simulink model "controller"  (R2022b)
settings: Solver=VariableStepAuto  StartTime=0.0  StopTime=160  RelTol=1e-3
undefined symbols (not defined in the file or in its folder): SS_glide_A, SS_glide_B, SS_glide_C, SS_glide_D
libraries: simulink_extras x5, cstblocks x2
settings Model: Creator=micky  LastModifiedBy=micky

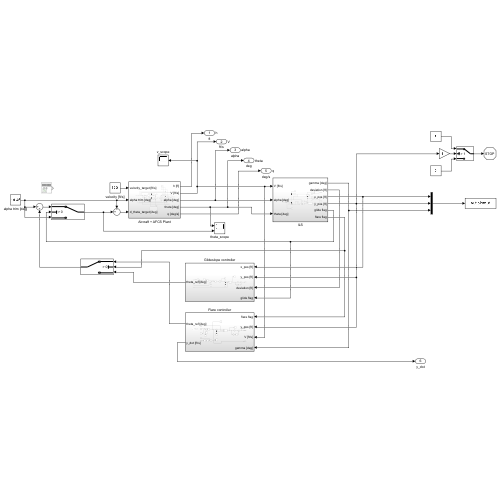
[thumbnail: Simulink's stored preview of the top-level diagram]
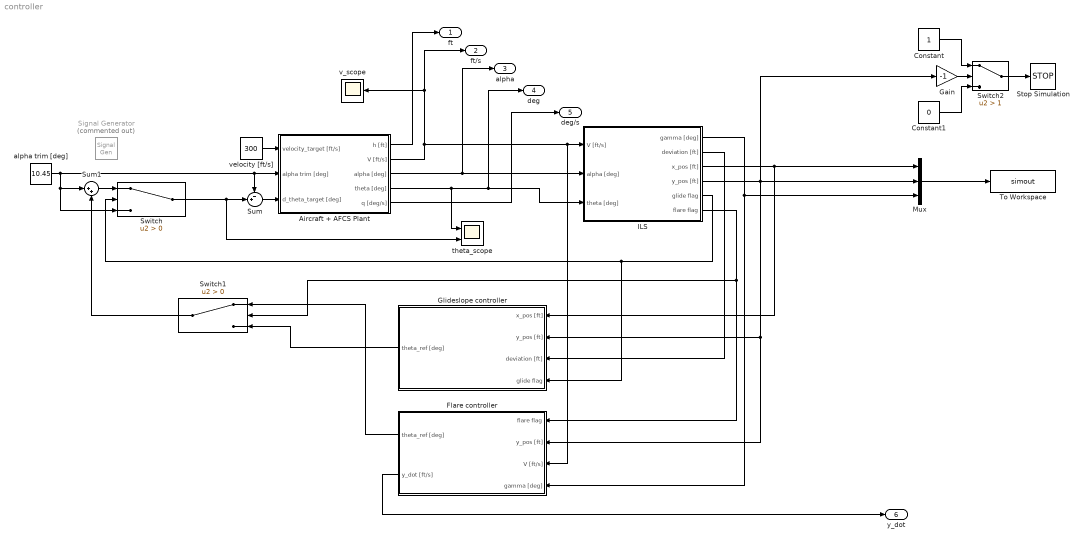
== system controller ==
  Aircraft + AFCS Plant : Subsystem
  Constant : Constant
  Constant1 : Constant  Value=0
  Flare controller : Subsystem
  Gain : Gain  Gain=-1
  Glideslope controller : Subsystem
  ILS : Subsystem
  Mux : Mux  Inputs=3
  Signal Generator : SignalGenerator  Commented=on  WaveForm=square  Frequency=0.6  Units=rad/sec
  Stop Simulation : Stop
  Sum : Sum  Inputs=-+|
  Sum1 : Sum  Inputs=|++
  Switch : Switch  Criteria=u2 > Threshold  SaturateOnIntegerOverflow=off  InputSameDT=off
  Switch1 : Switch  Criteria=u2 > Threshold  SaturateOnIntegerOverflow=off  InputSameDT=off
  Switch2 : Switch  Criteria=u2 > Threshold  Threshold=1  SaturateOnIntegerOverflow=off  InputSameDT=off
  To Workspace : ToWorkspace  VariableName=simout  SaveFormat=Timeseries  SampleTime=-1
  alpha trim [deg] : Constant  Value=10.45
  theta_scope : Scope  NumInputPorts=2
  v_scope : Scope
  velocity [ft/s] : Constant  Value=300
  ft : Outport  SignalName=h
  ft/s : Outport  Port=2  SignalName=V
  alpha : Outport  Port=3  SignalName=alpha
  deg : Outport  Port=4  SignalName=theta
  deg/s : Outport  Port=5  SignalName=q
  y_dot : Outport  Port=6
  wires:
  Aircraft + AFCS Plant/1(h [ft]) -> ft/1
  Aircraft + AFCS Plant/2(V [ft/s]) -> ft/s/1, v_scope/1, ILS/1(V [ft/s]), Flare controller/3(V [ft/s])
  Aircraft + AFCS Plant/3(alpha [deg]) -> alpha/1, ILS/2(alpha [deg])
  Aircraft + AFCS Plant/4(theta [deg]) -> theta_scope/1, ILS/3(theta [deg]), deg/1
  Aircraft + AFCS Plant/5(q [deg/s]) -> deg/s/1
  velocity [ft/s]/1 -> Aircraft + AFCS Plant/1(velocity_target [ft/s])
  ILS/1(gamma [deg]) -> Flare controller/4(gamma [deg]), Mux/3
  ILS/4(y_pos [ft]) -> Gain/1, Mux/2, Glideslope controller/2(y_pos [ft]), Flare controller/2(y_pos [ft])
  ILS/3(x_pos [ft]) -> Glideslope controller/1(x_pos [ft]), Mux/1
  ILS/2(deviation [ft]) -> Glideslope controller/3(deviation [ft])
  alpha trim [deg]/1 -> Sum/1, Aircraft + AFCS Plant/2(alpha trim [deg]), Sum1/1, Switch/3
  Glideslope controller/1(theta_ref [deg]) -> Switch1/3
  Sum/1 -> Aircraft + AFCS Plant/3(d_theta_target [deg])
  Switch/1 -> theta_scope/2, Sum/2
  Mux/1 -> To Workspace/1
  Switch1/1 -> Sum1/2
  Flare controller/1(theta_ref [deg]) -> Switch1/1
  ILS/5(glide flag) -> Glideslope controller/4(glide flag), Switch/2
  ILS/6(flare flag) -> Switch1/2, Flare controller/1(flare flag)
  Gain/1 -> Switch2/2
  Constant/1 -> Switch2/1
  Constant1/1 -> Switch2/3
  Switch2/1 -> Stop Simulation/1
  Flare controller/2(y_dot [ft/s]) -> y_dot/1
  Sum1/1 -> Switch/1

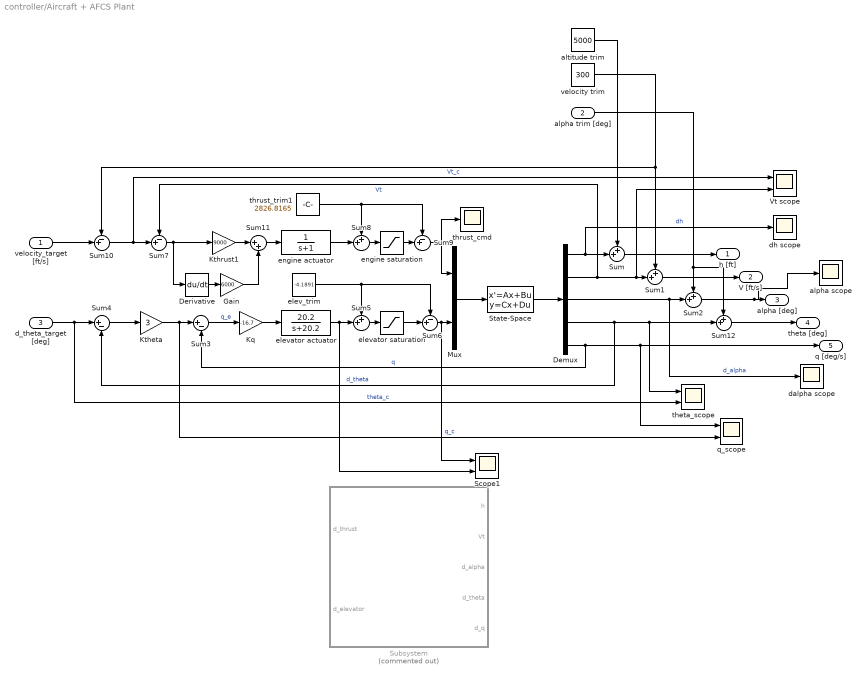
== system controller/Aircraft + AFCS Plant ==
  velocity_target [ft/s] : Inport
  alpha trim [deg] : Inport  Port=2
  d_theta_target [deg] : Inport  Port=3
  Demux : Demux  Outputs=5
  Derivative : Derivative
  Gain : Gain  Gain=6000
  Kq : Gain  Gain=-16.7
  Ktheta : Gain  Gain=3
  Kthrust1 : Gain  Gain=9000
  Mux : Mux  Inputs=2
  Scope1 : Scope  NumInputPorts=2
  State-Space : StateSpace  A=SS_glide_A  B=SS_glide_B  C=SS_glide_C  D=SS_glide_D  InitialCondition=0
  Subsystem : Subsystem  Commented=on
  Sum{,1..2,5,8,12} (6 alike) : Sum  Inputs=++|
  Sum{6..7,9..10} (4 alike) : Sum  Inputs=-+|
  Sum11 : Sum  Inputs=|++
  Sum3 : Sum  Inputs=|+-
  Sum4 : Sum  Inputs=|+-
  Vt scope : Scope  NumInputPorts=2
  alpha scope : Scope
  altitude trim : Constant  Value=5000
  dalpha scope : Scope
  dh scope : Scope
  elev_trim : Constant  Value=-4.1891
  elevator actuator : TransferFcn  Numerator=[20.2]  Denominator=[1 20.2]
  elevator saturation : Saturate  UpperLimit=25  LowerLimit=-25
  engine actuator : TransferFcn  Denominator=[1 1]
  engine saturation : Saturate  UpperLimit=19000  LowerLimit=1000
  q_scope : Scope  NumInputPorts=2
  theta_scope : Scope  NumInputPorts=2
  thrust_cmd : Scope
  thrust_trim1 : Constant  Value=2826.8165
  velocity trim : Constant  Value=300
  h [ft] : Outport
  V [ft/s] : Outport  Port=2
  alpha [deg] : Outport  Port=3
  theta [deg] : Outport  Port=4
  q [deg/s] : Outport  Port=5
  wires:
  engine actuator/1 -> Sum8/2
  Sum1/1 -> V [ft/s]/1
  Demux/5 -> Sum3/2, q [deg/s]/1, q_scope/1  "q"
  thrust_trim1/1 -> Sum9/1, Sum8/1
  Sum3/1 -> Kq/1  "q_e"
  Gain/1 -> Sum11/2
  Sum6/1 -> Scope1/1, Mux/2
  velocity_target [ft/s]/1 -> Sum10/2
  altitude trim/1 -> Sum/1
  Demux/3 -> dalpha scope/1, Sum2/2  "d_alpha"
  Kthrust1/1 -> Sum11/1
  Demux/2 -> Vt scope/2, Sum1/2, Sum7/1  "Vt"
  velocity trim/1 -> Sum10/1, Sum1/1
  Sum/1 -> h [ft]/1
  Sum10/1 -> Sum7/2, Vt scope/1  "Vt_c"
  State-Space/1 -> Demux/1
  Demux/4 -> Sum12/2, theta_scope/1, Sum4/2  "d_theta"
  Demux/1 -> dh scope/1, Sum/2  "dh"
  elev_trim/1 -> Sum6/1, Sum5/1
  Mux/1 -> State-Space/1
  Sum7/1 -> Kthrust1/1, Derivative/1
  Ktheta/1 -> q_scope/2, Sum3/1  "q_c"
  Sum4/1 -> Ktheta/1
  d_theta_target [deg]/1 -> theta_scope/2, Sum4/1  "theta_c"
  Sum2/1 -> alpha scope/1, alpha [deg]/1
  Sum5/1 -> elevator saturation/1
  Sum9/1 -> thrust_cmd/1, Mux/1
  Derivative/1 -> Gain/1
  engine saturation/1 -> Sum9/2
  Sum8/1 -> engine saturation/1
  elevator saturation/1 -> Sum6/2
  Kq/1 -> elevator actuator/1
  elevator actuator/1 -> Scope1/2, Sum5/2
  Sum11/1 -> engine actuator/1
  Sum12/1 -> theta [deg]/1
  alpha trim [deg]/1 -> Sum12/1, Sum2/1

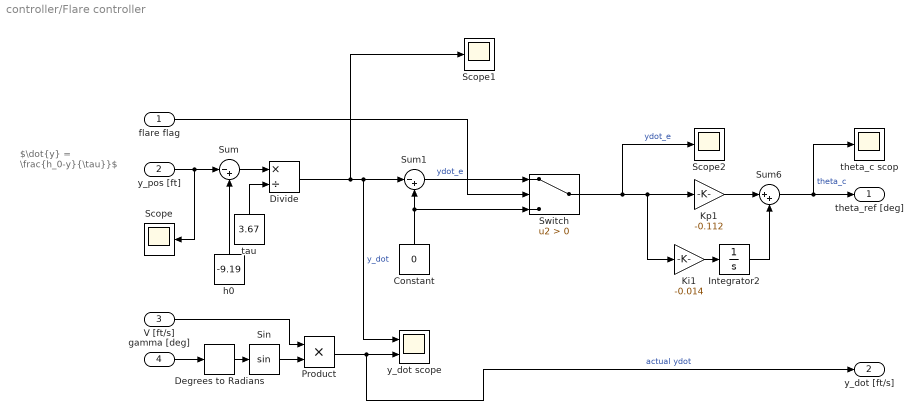
== system controller/Flare controller ==
  note: $\dot{y} = \frac{h_0-y}{\tau}}$
  flare flag : Inport
  y_pos [ft] : Inport  Port=2
  V [ft/s] : Inport  Port=3
  gamma [deg] : Inport  Port=4
  Constant : Constant  Value=0
  Degrees to Radians : simulink_extras/Transformations/Degrees to Radians
  Divide : Product  Inputs=*/
  Integrator2 : Integrator
  Ki1 : Gain  Gain=-0.014
  Kp1 : Gain  Gain=-0.112
  Product : Product
  Scope : Scope
  Scope1 : Scope
  Scope2 : Scope
  Sin : Trigonometry
  Sum : Sum  Inputs=|-+
  Sum1 : Sum  Inputs=|-+
  Sum6 : Sum  Inputs=|++
  Switch : Switch  Criteria=u2 > Threshold  SaturateOnIntegerOverflow=off  InputSameDT=off
  h0 : Constant  Value=-9.19
  tau : Constant  Value=3.67
  theta_c scop : Scope
  y_dot scope : Scope  NumInputPorts=2
  theta_ref [deg] : Outport
  y_dot [ft/s] : Outport  Port=2
  wires:
  h0/1 -> Sum/2
  y_pos [ft]/1 -> Sum/1, Scope/1
  Sum/1 -> Divide/1
  tau/1 -> Divide/2
  Divide/1 -> Scope1/1, Sum1/1, y_dot scope/1  "y_dot"
  gamma [deg]/1 -> Degrees to Radians/1
  Degrees to Radians/1 -> Sin/1
  Sin/1 -> Product/2
  V [ft/s]/1 -> Product/1
  Product/1 -> y_dot [ft/s]/1, y_dot scope/2  "actual ydot"
  Sum1/1 -> Switch/1  "ydot_e"
  Sum6/1 -> theta_c scop/1, theta_ref [deg]/1  "theta_c"
  Kp1/1 -> Sum6/1
  Switch/1 -> Scope2/1, Kp1/1, Ki1/1  "ydot_e"
  Ki1/1 -> Integrator2/1
  flare flag/1 -> Switch/2
  Constant/1 -> Switch/3, Sum1/2
  Integrator2/1 -> Sum6/2

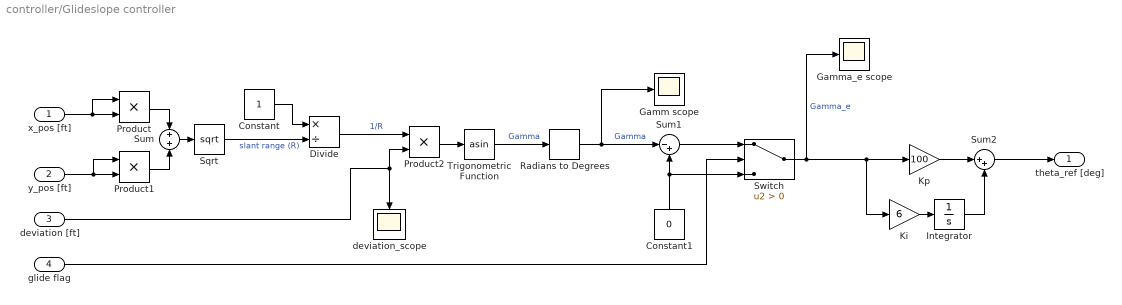
== system controller/Glideslope controller ==
  x_pos [ft] : Inport
  y_pos [ft] : Inport  Port=2
  deviation [ft] : Inport  Port=3
  glide flag : Inport  Port=4
  Constant : Constant
  Constant1 : Constant  Value=0
  Divide : Product  Inputs=*/
  Gamm scope : Scope
  Gamma_e scope : Scope
  Integrator : Integrator
  Ki : Gain  Gain=6
  Kp : Gain  Gain=100
  Product : Product
  Product1 : Product
  Product2 : Product
  Radians to Degrees : simulink_extras/Transformations/Radians to Degrees
  Sqrt : Sqrt
  Sum : Sum
  Sum1 : Sum  Inputs=|-+
  Sum2 : Sum  Inputs=|++
  Switch : Switch  Criteria=u2 > Threshold  SaturateOnIntegerOverflow=off  InputSameDT=off
  Trigonometric Function : Trigonometry  Operator=asin
  deviation_scope : Scope
  theta_ref [deg] : Outport
  wires:
  x_pos [ft]/1 -> Product/2, Product/1
  y_pos [ft]/1 -> Product1/1, Product1/2
  Product/1 -> Sum/1
  Product1/1 -> Sum/2
  Sum/1 -> Sqrt/1
  Sqrt/1 -> Divide/2  "slant range (R)"
  Constant/1 -> Divide/1
  Divide/1 -> Product2/1  "1/R"
  deviation [ft]/1 -> Product2/2, deviation_scope/1
  Product2/1 -> Trigonometric Function/1
  Switch/1 -> Kp/1, Ki/1, Gamma_e scope/1  "Gamma_e"
  Kp/1 -> Sum2/1
  Ki/1 -> Integrator/1
  Integrator/1 -> Sum2/2
  Sum2/1 -> theta_ref [deg]/1
  Radians to Degrees/1 -> Gamm scope/1, Sum1/1  "Gamma"
  glide flag/1 -> Switch/2
  Constant1/1 -> Switch/3, Sum1/2
  Sum1/1 -> Switch/1
  Trigonometric Function/1 -> Radians to Degrees/1  "Gamma"

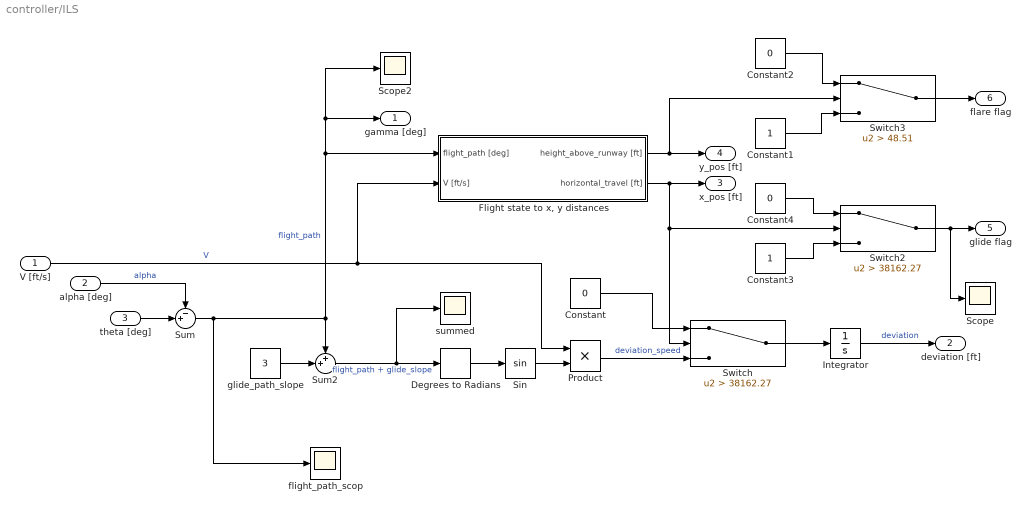
== system controller/ILS ==
  V [ft/s] : Inport
  alpha [deg] : Inport  Port=2
  theta [deg] : Inport  Port=3
  Constant : Constant  Value=0
  Constant1 : Constant
  Constant2 : Constant  Value=0
  Constant3 : Constant
  Constant4 : Constant  Value=0
  Degrees to Radians : simulink_extras/Transformations/Degrees to Radians
  "Flight state to x, y distances" : Subsystem
  Integrator : Integrator
  Product : Product
  Scope : Scope
  Scope2 : Scope
  Sin : Trigonometry
  Sum : Sum  Inputs=-+|
  Sum2 : Sum  Inputs=++|
  Switch : Switch  Criteria=u2 > Threshold  Threshold=38162.27  SaturateOnIntegerOverflow=off  InputSameDT=off
  Switch2 : Switch  Criteria=u2 > Threshold  Threshold=38162.27  SaturateOnIntegerOverflow=off  InputSameDT=off
  Switch3 : Switch  Criteria=u2 > Threshold  Threshold=48.51  SaturateOnIntegerOverflow=off  InputSameDT=off
  flight_path_scop : Scope
  glide_path_slope : Constant  Value=3
  summed : Scope
  gamma [deg] : Outport
  deviation [ft] : Outport  Port=2
  x_pos [ft] : Outport  Port=3
  y_pos [ft] : Outport  Port=4
  glide flag : Outport  Port=5
  flare flag : Outport  Port=6
  wires:
  glide_path_slope/1 -> Sum2/2
  V [ft/s]/1 -> Product/1, "Flight state to x, y distances"/2(V [ft/s])  "V"
  Degrees to Radians/1 -> Sin/1
  Sum/1 -> Sum2/1, Scope2/1, gamma [deg]/1, "Flight state to x, y distances"/1(flight_path [deg]), flight_path_scop/1  "flight_path"
  Sum2/1 -> summed/1, Degrees to Radians/1  "flight_path + glide_slope"
  Integrator/1 -> deviation [ft]/1  "deviation"
  Product/1 -> Switch/3  "deviation_speed"
  Sin/1 -> Product/2
  alpha [deg]/1 -> Sum/1  "alpha"
  theta [deg]/1 -> Sum/2
  Constant/1 -> Switch/1
  Switch/1 -> Integrator/1
  Switch2/1 -> Scope/1, glide flag/1
  Constant1/1 -> Switch3/3
  Constant2/1 -> Switch3/1
  Constant4/1 -> Switch2/1
  Constant3/1 -> Switch2/3
  Switch3/1 -> flare flag/1
  "Flight state to x, y distances"/2(horizontal_travel [ft]) -> x_pos [ft]/1, Switch/2, Switch2/2
  "Flight state to x, y distances"/1(height_above_runway [ft]) -> y_pos [ft]/1, Switch3/2

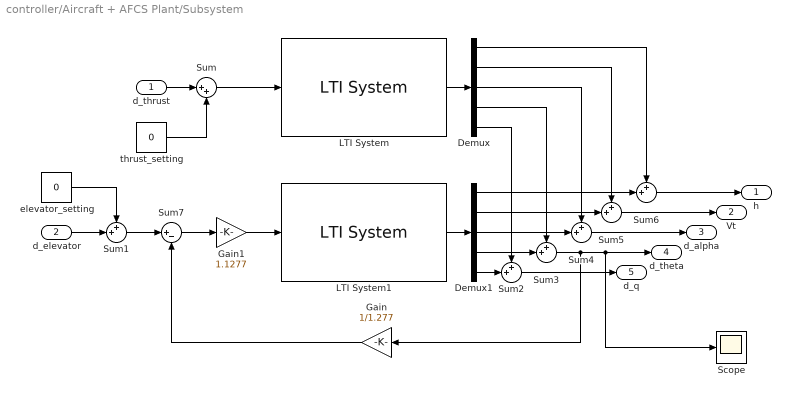
== system controller/Aircraft + AFCS Plant/Subsystem ==
  d_thrust : Inport
  d_elevator : Inport  Port=2
  Demux : Demux  Outputs=5
  Demux1 : Demux  Outputs=5
  Gain : Gain  Gain=1/1.277
  Gain1 : Gain  Gain=1.1277
  LTI System : cstblocks/LTI System  sys=thrust_2_outs  IC=[]
  LTI System1 : cstblocks/LTI System  sys=elevator_2_outs  IC=[]
  Scope : Scope
  Sum : Sum  Inputs=|++
  Sum{1..6} (6 alike) : Sum  Inputs=++|
  Sum7 : Sum  Inputs=|+-
  elevator_setting : Constant  Value=0
  thrust_setting : Constant  Value=0
  h : Outport
  Vt : Outport  Port=2
  d_alpha : Outport  Port=3
  d_theta : Outport  Port=4
  d_q : Outport  Port=5
  wires:
  LTI System/1 -> Demux/1
  LTI System1/1 -> Demux1/1
  Demux1/5 -> Sum2/2
  Sum2/1 -> d_q/1
  Sum3/1 -> Gain/1, Scope/1, d_theta/1
  Demux1/4 -> Sum3/2
  Sum4/1 -> d_alpha/1
  Demux1/3 -> Sum4/2
  Sum5/1 -> Vt/1
  Demux1/2 -> Sum5/2
  Sum6/1 -> h/1
  Demux1/1 -> Sum6/2
  Demux/5 -> Sum2/1
  Demux/4 -> Sum3/1
  Demux/3 -> Sum4/1
  Demux/2 -> Sum5/1
  Demux/1 -> Sum6/1
  d_elevator/1 -> Sum1/2
  d_thrust/1 -> Sum/1
  Sum/1 -> LTI System/1
  thrust_setting/1 -> Sum/2
  elevator_setting/1 -> Sum1/1
  Gain/1 -> Sum7/2
  Gain1/1 -> LTI System1/1
  Sum1/1 -> Sum7/1
  Sum7/1 -> Gain1/1

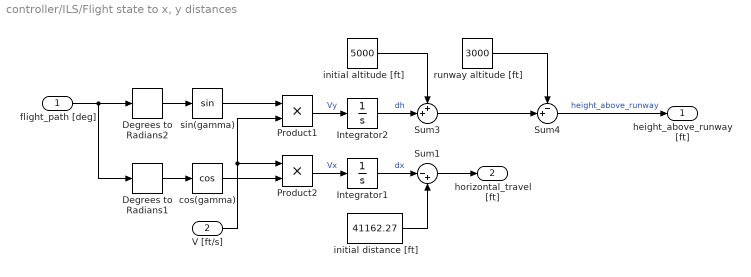
== system controller/ILS/Flight state to x, y distances ==
  flight_path [deg] : Inport
  V [ft/s] : Inport  Port=2
  Degrees to Radians1 : simulink_extras/Transformations/Degrees to Radians
  Degrees to Radians2 : simulink_extras/Transformations/Degrees to Radians
  Integrator1 : Integrator
  Integrator2 : Integrator
  Product1 : Product
  Product2 : Product
  Sum1 : Sum  Inputs=|-+
  Sum3 : Sum  Inputs=++|
  Sum4 : Sum  Inputs=-+|
  cos(gamma) : Trigonometry  Operator=cos
  initial altitude [ft] : Constant  Value=5000
  initial distance [ft] : Constant  Value=41162.27
  runway altitude [ft] : Constant  Value=3000
  sin(gamma) : Trigonometry
  height_above_runway [ft] : Outport
  horizontal_travel [ft] : Outport  Port=2
  wires:
  Sum1/1 -> horizontal_travel [ft]/1
  Product2/1 -> Integrator1/1  "Vx"
  Product1/1 -> Integrator2/1  "Vy"
  Integrator2/1 -> Sum3/2  "dh"
  Degrees to Radians1/1 -> cos(gamma)/1
  Sum3/1 -> Sum4/2
  Integrator1/1 -> Sum1/1  "dx"
  Sum4/1 -> height_above_runway [ft]/1  "height_above_runway"
  initial altitude [ft]/1 -> Sum3/1
  Degrees to Radians2/1 -> sin(gamma)/1
  runway altitude [ft]/1 -> Sum4/1
  initial distance [ft]/1 -> Sum1/2
  sin(gamma)/1 -> Product1/1
  V [ft/s]/1 -> Product1/2, Product2/1
  cos(gamma)/1 -> Product2/2
  flight_path [deg]/1 -> Degrees to Radians1/1, Degrees to Radians2/1
